simulink model "D24P414_1_model02"  (R2021a)
settings: Solver=VariableStepAuto  StartTime=0.0  StopTime=7  FixedStep=1e-6  RelTol=1e-3
values from neighbouring files (symbols this model uses):
  p_ic = climate_p    [D24P414_1_script.m]
  params_fruit = fruit_p    [D24P414_1_script.m]
  t0_shift = days(t0-t0_12_00)    [D24P414_1_script.m]
  x0_fruit = fruit_ic    [D24P414_1_script.m]
  x0_ic = climate_ic    [D24P414_1_script.m]
libraries: HORTISIM x14
(part 1 of 2)
settings Model: SimulationMode=accelerator  Creator=djoroya  LastModifiedBy=djoroya
settings SolverCC: MaxConsecutiveZCs=100  MaxConsecutiveMinStep=5
settings DebuggingCC: UnconnectedInputMsg=none  UnconnectedOutputMsg=none  UnconnectedLineMsg=none
settings HardwareCC: TargetBitPerLong=64  TargetBitPerPointer=64  TargetBitPerSizeT=64  TargetBitPerPtrDiffT=64  TargetLongLongMode=on  TargetIntDivRoundTo=Zero  TargetEndianess=LittleEndian  TargetWordSize=64  TargetHWDeviceType=MATLAB Host  ProdEqTarget=off
settings RTWCC: Description=Rapid Simulation Target  SystemTargetFile=rsim.tlc  TemplateMakefile=rsim_default_tmf
settings RSimTargetCC: TargetLangStandard=C99 (ISO)

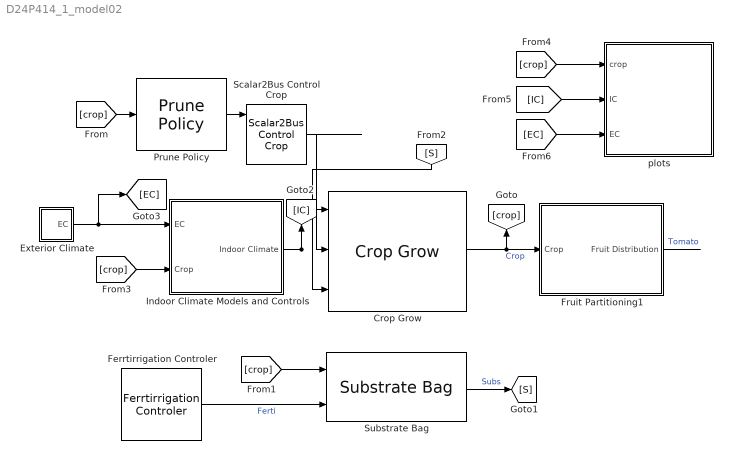
== system D24P414_1_model02 ==
  Crop Grow : HORTISIM/Horticulture/Models/Crop Grow  params=crop_params  x0=x0_crop
      settings: SourceProductName=Horti Simulator
  Exterior Climate : Subsystem
  Ferrtirrigation Controler : HORTISIM/Horticulture/Controls/Ferrtirrigation  Controler  SystemSampleTime=-1  VariantActivationTime=update diagram  Latency=0  AutoFrameSizeCalculation=off
      settings: SourceProductName=Horti Simulator
  Fruit Partitioning1 : Subsystem  AncestorBlock=HORTISIM/Horticulture/Models/Fruit Partitioning1  mask{x0=x0_fruit, params=params_fruit}
      mask Display: image('$imagefile'); % Use "Edit Image" on toolstrip to change.
  Indoor Climate Models and Controls : Subsystem
  Prune Policy : HORTISIM/Horticulture/Controls/Prune Policy  SystemSampleTime=-1  VariantActivationTime=update diagram  Latency=0  AutoFrameSizeCalculation=off
      settings: SourceProductName=Horti Simulator
  Scalar2Bus Control Crop : HORTISIM/Other  Functions/Scalar2Bus Control Crop  SystemSampleTime=-1  VariantActivationTime=update diagram  Latency=0  AutoFrameSizeCalculation=off
      settings: SourceProductName=Horti Simulator
  Substrate Bag : HORTISIM/Horticulture/Models/Substrate Bag  x0=x0_substrate  params=substrate_params
      settings: SourceProductName=Horti Simulator
  plots : Subsystem
  wires:
  Exterior Climate/1(EC) -> [EC], Indoor Climate Models and Controls/1(EC)
  Indoor Climate Models and Controls/1(Indoor Climate) -> [IC], Crop Grow/1
  Crop Grow/1 -> [crop], Fruit Partitioning1/1(Crop)  "Crop"
  Ferrtirrigation Controler/1 -> Substrate Bag/2  "Ferti"
  Scalar2Bus Control Crop/1 -> Crop Grow/2
  Prune Policy/1 -> Scalar2Bus Control Crop/1
  [crop] -> Prune Policy/1
  [crop] -> Substrate Bag/1
  Substrate Bag/1 -> [S]  "Subs"
  [S] -> Crop Grow/3
  [crop] -> Indoor Climate Models and Controls/2(Crop)
  Fruit Partitioning1/1(Fruit Distribution) -> ?  "Tomato"
  [crop] -> plots/1(crop)
  [IC] -> plots/2(IC)
  [EC] -> plots/3(EC)

== system D24P414_1_model02/Exterior Climate ==
  Demux : Demux
  From Workspace : FromWorkspace  VariableName=EC
  Scalar2Bus External Climate : HORTISIM/Other  Functions/Scalar2Bus External Climate  SystemSampleTime=-1  VariantActivationTime=update diagram  Latency=0  AutoFrameSizeCalculation=off
      settings: SourceProductName=Horti Simulator
  EC : Outport
  wires:
  Demux/3 -> Scalar2Bus External Climate/3
  Demux/2 -> Scalar2Bus External Climate/2
  Scalar2Bus External Climate/1 -> EC/1
  Demux/1 -> Scalar2Bus External Climate/1
  Demux/4 -> Scalar2Bus External Climate/4
  From Workspace/1 -> Demux/1

== system D24P414_1_model02/Fruit Partitioning1 ==
  In Bus Element : Inport  PortName=Crop  Element=Tsum
  In Bus Element1 : Inport  PortName=Crop  Element=HeatVars.TvegMean
  In Bus Element3 : Inport  PortName=Crop  Element=plants_density
  In Bus Element4 : Inport  PortName=Crop  Element=Carbon.Cfruit
  Integrator : Integrator  InitialCondition=1e-3
  MATLAB Function : MATLAB Function  TreatAsAtomicUnit=on
  Scope : Scope  NumInputPorts=2
  Scope1 : Scope
  Fruit Distribution : Outport
  wires:
  MATLAB Function/2(DT) -> Scope1/1
  In Bus Element1/1 -> MATLAB Function/4(T)
  Integrator/1 -> Scope/2, Fruit Distribution/1, MATLAB Function/3(Cfruit_mature)
  MATLAB Function/1(dCmdt) -> Integrator/1
  In Bus Element/1 -> MATLAB Function/2(Tsum)
  In Bus Element4/1 -> MATLAB Function/1(Cfruit), Scope/1

== system D24P414_1_model02/Indoor Climate Models and Controls ==
  EC : Inport
  Crop : Inport  Port=2
  Climate Model : Subsystem  Variant=on  VariantControlMode=label  VariantControl=Choice  LabelModeActiveChoice=Choice
  Control System : Subsystem
      settings: PortSchema="{\"entries\":[{\"content\":{\"sides\":[{\"content\":{\"connectorIds\":[\"In1\",\"In2\",\"In3\"]},\"type\":\"ConnectorPlacement.EquallySpacedRectSide\",\"uuid\":\"7d0146e2-a53b-49ab-a7f4-04cd7ef00b9a\"},{\"content\":{\"connectorIds\":[\"Out1\",\"Out2\"],\"side\":\"RIGHT\"},\"type\":\"ConnectorPlacement.EquallySpacedRectSide\",\"uuid\":\"fee587e2-4b5c-4140-8904-07609d427593\"},{\"content\":{\"connectorIds\":[],\"side\":\"TOP\"},\"type\":\"ConnectorPlacement.EquallySpacedRectSide\",\"uuid\":\"52e767bc-1595-40ac-996f-44c9eedd0a08\"},{\"content\":{\"connectorIds\":[\"In4\"],\"side\":\"BOTTOM\"},\"type\":\"ConnectorPlacement.EquallySpacedRectSide\",\"uuid\":\"c629db5c-cfe6-4bd1-aeb9-7fba46dde396\"}]},\"type\":\"ConnectorPlacement.EquallySpacedConnector\",\"uuid\":\"268fde01-3c08-4d62-bfbb-fc94284c5cdd\"}],\"packageUris\":[\"http://schema.mathworks.com/mf0/Connector/R2020b\"],\"version\":\"1.0\"}"
  Set Point Controler : Subsystem
      settings: PortSchema="{\"entries\":[{\"content\":{\"sides\":[{\"content\":{\"connectorIds\":[\"Out1\",\"In1\"]},\"type\":\"ConnectorPlacement.EquallySpacedRectSide\",\"uuid\":\"f4e16d49-2d4b-4271-89b5-3d9d4afc6df8\"},{\"content\":{\"connectorIds\":[],\"side\":\"RIGHT\"},\"type\":\"ConnectorPlacement.EquallySpacedRectSide\",\"uuid\":\"2cc2085b-d4b5-43d5-9499-e0c517c8a674\"},{\"content\":{\"connectorIds\":[],\"side\":\"TOP\"},\"type\":\"ConnectorPlacement.EquallySpacedRectSide\",\"uuid\":\"ad83e959-9e1e-4ed4-97a9-5adb1e75d698\"},{\"content\":{\"connectorIds\":[\"In2\"],\"side\":\"BOTTOM\"},\"type\":\"ConnectorPlacement.EquallySpacedRectSide\",\"uuid\":\"c1e716b8-742f-4738-a087-b5d9edc55981\"}]},\"type\":\"ConnectorPlacement.EquallySpacedConnector\",\"uuid\":\"8204d6bf-0a3a-4b44-b0bf-e9541e9654ff\"}],\"packageUris\":[\"http://schema.mathworks.com/mf0/Connector/R2020b\"],\"version\":\"1.0\"}"
  Indoor Climate : Outport
  wires:
  EC/1 -> Climate Model/3(EC), Control System/4(EC), Set Point Controler/2(EC)
  Crop/1 -> Control System/3(Crop), Set Point Controler/1(Crop)
  Set Point Controler/1(ST) -> Control System/2(ST)
  Control System/1(Ext) -> Climate Model/1(Ext)
  Control System/2(CoCl1) -> Climate Model/2(Control)  "Control"
  Climate Model/1(Climate) -> Control System/1(IC), Indoor Climate/1  "Indoor Climate"

== system D24P414_1_model02/plots ==
  crop : Inport
  IC : Inport  Port=2
  EC : Inport  Port=3
  Bus Selector : BusSelector  OutputSignals=Carbon.Cbuff,Carbon.Cfruit,Carbon.Cleaf,Carbon.Cstem
  Bus Selector1 : BusSelector  OutputSignals=Temp.Tair,QS.R_int
  Heater : Subsystem
  Scope : Scope  NumInputPorts=4
  Windows : Subsystem
  tag scope: R=global
  wires:
  Bus Selector/4 -> Scope/4  "<Cstem>"
  Bus Selector/3 -> Scope/3  "<Cleaf>"
  Bus Selector/2 -> Scope/2  "<Cfruit>"
  Bus Selector/1 -> Scope/1  "<Cbuff>"
  crop/1 -> Bus Selector/1
  IC/1 -> Bus Selector1/1
  Bus Selector1/2 -> [R]  "<R_int>"
  EC/1 -> Windows/1(In1), Heater/1(EC)
  Bus Selector1/1 -> Heater/2(<Tair>), Windows/2(<Tair>)  "<Tair>"

== system D24P414_1_model02/Indoor Climate Models and Controls/Climate Model ==
  Ext : Inport
  Control : Inport  Port=2
  EC : Inport  Port=3
  Climate Model : Subsystem  AncestorBlock=HORTISIM/Climate/Models/Climate Model  VariantControl=Choice  mask{params=p_ic, x0=x0_ic}
      mask Display: image('$imagefile'); % Use "Edit Image" on toolstrip to change.
  Climate : Outport

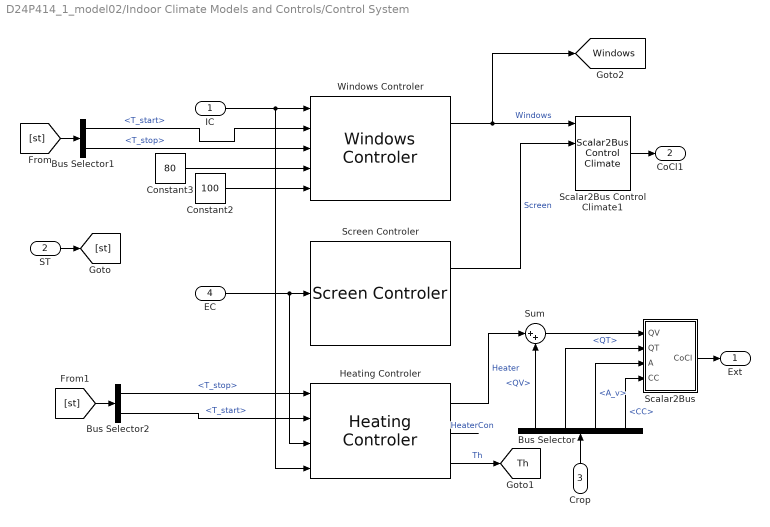
== system D24P414_1_model02/Indoor Climate Models and Controls/Control System ==
  IC : Inport
  ST : Inport  Port=2
  Crop : Inport  Port=3
  EC : Inport  Port=4
  Bus Selector : BusSelector  OutputSignals=HeatVars.QV,HeatVars.QT,A_v,CC
  Bus Selector1 : BusSelector  OutputSignals=Heater.T_start,Windows.T_stop
  Bus Selector2 : BusSelector  OutputSignals=Heater.T_stop,Heater.T_start
  Constant2 : Constant  Value=100
  Constant3 : Constant  Value=80
  Heating Controler : HORTISIM/Climate/Controls/Heating Controler  params=HP  x0=x0_H
      settings: SourceProductName=Horti Simulator
  "Scalar2Bus " : Subsystem
  Scalar2Bus Control Climate1 : HORTISIM/Other  Functions/Scalar2Bus  Control Climate  SystemSampleTime=-1  VariantActivationTime=update diagram  Latency=0  AutoFrameSizeCalculation=off
      settings: SourceProductName=Horti Simulator
  Screen Controler : HORTISIM/Climate/Controls/Screen Controler  params=scr_p
      settings: SourceProductName=Horti Simulator
  Sum : Sum  Inputs=|++
  Windows Controler : HORTISIM/Climate/Controls/Windows Controler  params=win_p
      settings: SourceProductName=Horti Simulator
  Ext : Outport
  CoCl1 : Outport  Port=2
  tag scope: Th=global, Windows=global
  wires:
  EC/1 -> Heating Controler/3, Screen Controler/1
  "Scalar2Bus "/1(CoCl) -> Ext/1
  Windows Controler/1 -> [Windows], Scalar2Bus Control Climate1/1  "Windows"
  Scalar2Bus Control Climate1/1 -> CoCl1/1
  Screen Controler/1 -> Scalar2Bus Control Climate1/2  "Screen"
  IC/1 -> Heating Controler/4, Windows Controler/1
  Constant2/1 -> Windows Controler/5
  Constant3/1 -> Windows Controler/4
  Bus Selector1/1 -> Windows Controler/2  "<T_start>"
  Bus Selector1/2 -> Windows Controler/3  "<T_stop>"
  Crop/1 -> Bus Selector/1
  Sum/1 -> "Scalar2Bus "/1(QV)
  Bus Selector/1 -> Sum/2  "<QV>"
  Heating Controler/1 -> Sum/1  "Heater"
  Bus Selector/2 -> "Scalar2Bus "/2(QT)  "<QT>"
  Bus Selector/3 -> "Scalar2Bus "/3(A)  "<A_v>"
  Bus Selector/4 -> "Scalar2Bus "/4(CC)  "<CC>"
  ST/1 -> [st]
  [st] -> Bus Selector1/1
  [st] -> Bus Selector2/1
  Heating Controler/3 -> [Th]  "Th"
  Heating Controler/2 -> ?  "HeaterCon"
  Bus Selector2/2 -> Heating Controler/2  "<T_start>"
  Bus Selector2/1 -> Heating Controler/1  "<T_stop>"

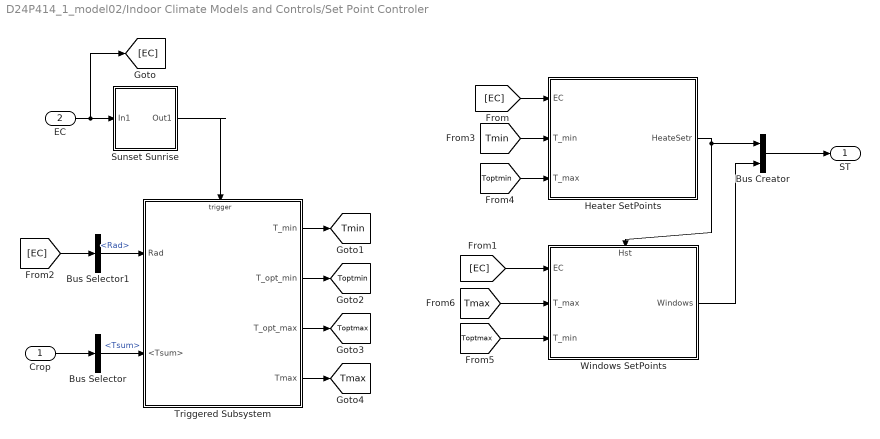
== system D24P414_1_model02/Indoor Climate Models and Controls/Set Point Controler ==
  Crop : Inport
  EC : Inport  Port=2
  Bus Creator : BusCreator  Inputs=2
  Bus Selector : BusSelector  OutputSignals=Tsum
  Bus Selector1 : BusSelector  OutputSignals=Rad
  Heater SetPoints : Subsystem
  Sunset Sunrise : Subsystem
  Triggered Subsystem : Subsystem  TreatAsAtomicUnit=on
  Windows SetPoints : Subsystem
      settings: PortSchema="{\"entries\":[{\"content\":{\"sides\":[{\"content\":{\"connectorIds\":[\"In1\",\"In2\",\"In3\"]},\"type\":\"ConnectorPlacement.EquallySpacedRectSide\",\"uuid\":\"adbf67af-74ef-4d44-a221-2fa9350c3df6\"},{\"content\":{\"connectorIds\":[\"Out1\"],\"side\":\"RIGHT\"},\"type\":\"ConnectorPlacement.EquallySpacedRectSide\",\"uuid\":\"184ab568-f69f-420e-aba1-0e27e090a144\"},{\"content\":{\"connectorIds\":[\"In4\"],\"side\":\"TOP\"},\"type\":\"ConnectorPlacement.EquallySpacedRectSide\",\"uuid\":\"ef86e682-f841-40e3-b028-22b4dc12532c\"}]},\"type\":\"ConnectorPlacement.EquallySpacedConnector\",\"uuid\":\"71dd7da4-de02-4916-9a1b-70690742187b\"}],\"packageUris\":[\"http://schema.mathworks.com/mf0/Connector/R2020b\"],\"version\":\"1.0\"}"
  ST : Outport
  tag scope: Tmax=global, Tmin=global, Toptmax=global, Toptmin=global
  wires:
  Bus Creator/1 -> ST/1
  Heater SetPoints/1(HeateSetr) -> Windows SetPoints/4(Hst), Bus Creator/1
  Windows SetPoints/1(Windows) -> Bus Creator/2
  Crop/1 -> Bus Selector/1
  Sunset Sunrise/1(Out1) -> Triggered Subsystem/Trigger
  EC/1 -> [EC], Sunset Sunrise/1(In1)
  Bus Selector/1 -> Triggered Subsystem/2(<Tsum>)  "<Tsum>"
  Bus Selector1/1 -> Triggered Subsystem/1(Rad)  "<Rad>"
  [EC] -> Heater SetPoints/1(EC)
  [EC] -> Windows SetPoints/1(EC)
  [EC] -> Bus Selector1/1
  Triggered Subsystem/2(T_opt_min) -> [Toptmin]
  Triggered Subsystem/4(Tmax) -> [Tmax]
  Triggered Subsystem/1(T_min) -> [Tmin]
  Triggered Subsystem/3(T_opt_max) -> [Toptmax]
  [Tmin] -> Heater SetPoints/2(T_min)
  [Toptmin] -> Heater SetPoints/3(T_max)
  [Toptmax] -> Windows SetPoints/3(T_min)
  [Tmax] -> Windows SetPoints/2(T_max)

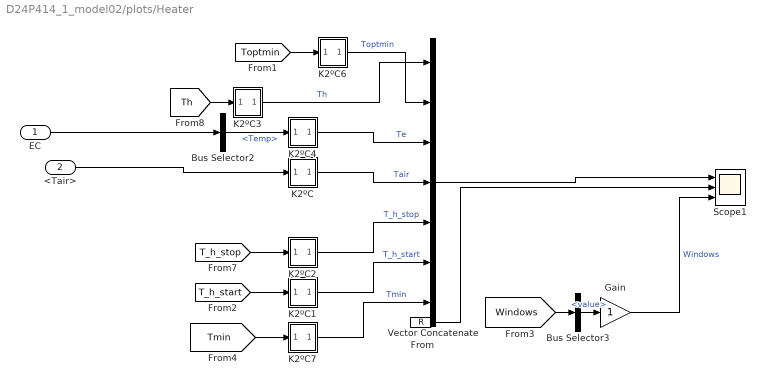
== system D24P414_1_model02/plots/Heater ==
  EC : Inport
  <Tair> : Inport  Port=2
  Bus Selector2 : BusSelector  OutputSignals=Temp
  Bus Selector3 : BusSelector  OutputSignals=value
  Gain : Gain
  K2ºC : Subsystem
  K2ºC1 : Subsystem
  K2ºC2 : Subsystem
  K2ºC3 : Subsystem
  K2ºC4 : Subsystem
  K2ºC6 : Subsystem
  K2ºC7 : Subsystem
  Scope1 : Scope  NumInputPorts=3
  Vector Concatenate : Concatenate  NumInputs=7
  wires:
  EC/1 -> Bus Selector2/1
  Bus Selector3/1 -> Gain/1  "<value>"
  [Toptmin] -> K2ºC6/1(In1)
  [R] -> Scope1/2
  K2ºC2/1(Out1) -> Vector Concatenate/5  "T_h_stop"
  Gain/1 -> Scope1/3  "Windows"
  Bus Selector2/1 -> K2ºC4/1(In1)  "<Temp>"
  K2ºC4/1(Out1) -> Vector Concatenate/3  "Te"
  [Tmin] -> K2ºC7/1(In1)
  [T_h_stop] -> K2ºC2/1(In1)
  <Tair>/1 -> K2ºC/1(In1)
  K2ºC7/1(Out1) -> Vector Concatenate/7  "Tmin"
  [Windows] -> Bus Selector3/1
  Vector Concatenate/1 -> Scope1/1
  K2ºC6/1(Out1) -> Vector Concatenate/2  "Toptmin"
  K2ºC/1(Out1) -> Vector Concatenate/4  "Tair"
  [T_h_start] -> K2ºC1/1(In1)
  K2ºC1/1(Out1) -> Vector Concatenate/6  "T_h_start"
  [Th] -> K2ºC3/1(In1)
  K2ºC3/1(Out1) -> Vector Concatenate/1  "Th"

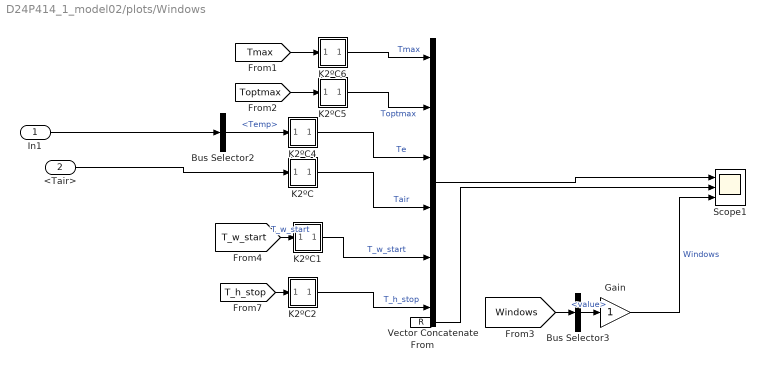
== system D24P414_1_model02/plots/Windows ==
  In1 : Inport
  <Tair> : Inport  Port=2
  Bus Selector2 : BusSelector  OutputSignals=Temp
  Bus Selector3 : BusSelector  OutputSignals=value
  Gain : Gain
  K2ºC : Subsystem
  K2ºC1 : Subsystem
  K2ºC2 : Subsystem
  K2ºC4 : Subsystem
  K2ºC5 : Subsystem
  K2ºC6 : Subsystem
  Scope1 : Scope  NumInputPorts=3
  Vector Concatenate : Concatenate  NumInputs=6
  wires:
  In1/1 -> Bus Selector2/1
  Bus Selector3/1 -> Gain/1  "<value>"
  [Toptmax] -> K2ºC5/1(In1)
  [Tmax] -> K2ºC6/1(In1)
  [R] -> Scope1/2
  K2ºC2/1(Out1) -> Vector Concatenate/6  "T_h_stop"
  K2ºC5/1(Out1) -> Vector Concatenate/2  "Toptmax"
  Gain/1 -> Scope1/3  "Windows"
  Bus Selector2/1 -> K2ºC4/1(In1)  "<Temp>"
  K2ºC4/1(Out1) -> Vector Concatenate/3  "Te"
  [T_h_stop] -> K2ºC2/1(In1)
  <Tair>/1 -> K2ºC/1(In1)
  [Windows] -> Bus Selector3/1
  Vector Concatenate/1 -> Scope1/1
  K2ºC6/1(Out1) -> Vector Concatenate/1  "Tmax"
  K2ºC/1(Out1) -> Vector Concatenate/4  "Tair"
  K2ºC1/1(Out1) -> Vector Concatenate/5  "T_w_start"
  [T_w_start] -> K2ºC1/1(In1)  "T_w_start"

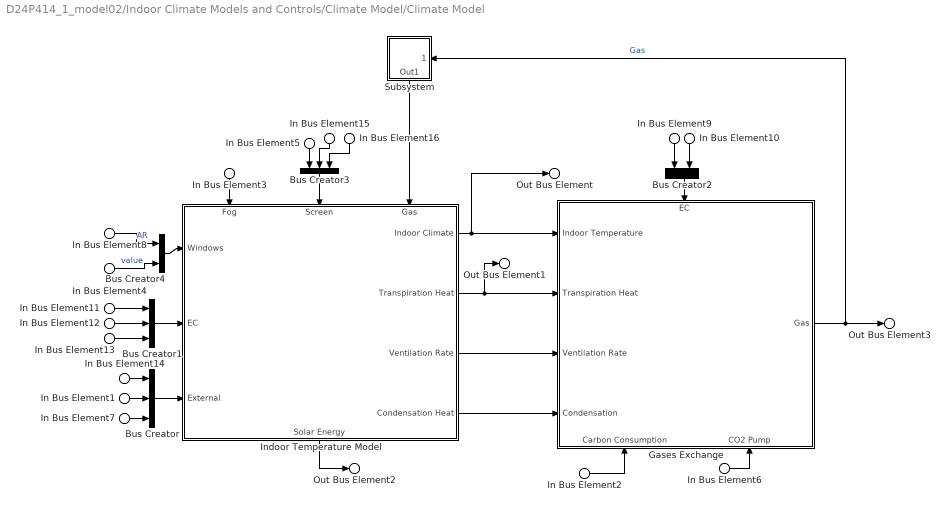
== system D24P414_1_model02/Indoor Climate Models and Controls/Climate Model/Climate Model ==
  In Bus Element14 : Inport  PortName=Ext  Element=QT
  In Bus Element1 : Inport  PortName=Ext  Element=QV
  In Bus Element2 : Inport  PortName=Ext  Element=CC
  In Bus Element7 : Inport  PortName=Ext  Element=A
  In Bus Element3 : Inport  Port=2  PortName=Control  Element=Fog
  In Bus Element5 : Inport  Port=2  PortName=Control  Element=Screen.gamma_max
  In Bus Element15 : Inport  Port=2  PortName=Control  Element=Screen.value
  In Bus Element16 : Inport  Port=2  PortName=Control  Element=Screen.beta
  In Bus Element6 : Inport  Port=2  PortName=Control  Element=CO2
  In Bus Element8 : Inport  Port=2  PortName=Control  Element=Windows.AR
  In Bus Element4 : Inport  Port=2  PortName=Control  Element=Windows.value
  In Bus Element9 : Inport  Port=3  PortName=EC  Element=HR
  In Bus Element10 : Inport  Port=3  PortName=EC  Element=Temp
  In Bus Element11 : Inport  Port=3  PortName=EC  Element=Temp
  In Bus Element12 : Inport  Port=3  PortName=EC  Element=Rad
  In Bus Element13 : Inport  Port=3  PortName=EC  Element=Wind
  Bus Creator : BusCreator  Inputs=3
  Bus Creator1 : BusCreator  Inputs=3
  Bus Creator2 : BusCreator  Inputs=2
  Bus Creator3 : BusCreator  Inputs=3
  Bus Creator4 : BusCreator  Inputs=2
  Gases Exchange : Subsystem
      settings: PortSchema="{\"entries\":[{\"content\":{\"sides\":[{\"content\":{\"connectorIds\":[\"In1\",\"In2\",\"In3\",\"In4\"]},\"type\":\"ConnectorPlacement.EquallySpacedRectSide\",\"uuid\":\"550da9a1-5f22-4db3-9ee3-e3750278f626\"},{\"content\":{\"connectorIds\":[\"Out1\"],\"side\":\"RIGHT\"},\"type\":\"ConnectorPlacement.EquallySpacedRectSide\",\"uuid\":\"cf559ec0-337d-42e7-96bb-a49ff9e682f6\"},{\"content\":{\"connectorIds\":[\"In5\"],\"side\":\"TOP\"},\"type\":\"ConnectorPlacement.EquallySpacedRectSide\",\"uuid\":\"d9874986-c35c-443c-9325-7a886074565b\"},{\"content\":{\"connectorIds\":[\"In6\",\"In7\"],\"side\":\"BOTTOM\"},\"type\":\"ConnectorPlacement.EquallySpacedRectSide\",\"uuid\":\"7f205c84-db2c-43a4-94ce-a6d2142a4e50\"}]},\"type\":\"ConnectorPlacement.EquallySpacedConnector\",\"uuid\":\"56c5cbc1-f580-43fc-9d79-62500ce9be4b\"}],\"packageUris\":[\"http://schema.mathworks.com/mf0/Connector/R2020b\"],\"version\":\"1.0\"}"
  Indoor Temperature Model : Subsystem
      settings: PortSchema="{\"entries\":[{\"content\":{\"sides\":[{\"content\":{\"connectorIds\":[\"In1\",\"In2\",\"In3\"]},\"type\":\"ConnectorPlacement.EquallySpacedRectSide\",\"uuid\":\"402556d7-b277-4cb3-8556-883bae99c69c\"},{\"content\":{\"connectorIds\":[\"Out1\",\"Out2\",\"Out3\",\"Out4\"],\"side\":\"RIGHT\"},\"type\":\"ConnectorPlacement.EquallySpacedRectSide\",\"uuid\":\"e8ec9f82-8759-4d98-a5e5-ef4db996ec8c\"},{\"content\":{\"connectorIds\":[\"In4\",\"In5\",\"In6\"],\"side\":\"TOP\"},\"type\":\"ConnectorPlacement.EquallySpacedRectSide\",\"uuid\":\"99d33cea-a089-4bcb-9505-68914c63f152\"},{\"content\":{\"connectorIds\":[\"Out5\"],\"side\":\"BOTTOM\"},\"type\":\"ConnectorPlacement.EquallySpacedRectSide\",\"uuid\":\"61ead6b3-0464-47f9-9f23-19f86056b325\"}]},\"type\":\"ConnectorPlacement.EquallySpacedConnector\",\"uuid\":\"a07dfd2f-7b40-4439-87f5-f093ac984b26\"}],\"packageUris\":[\"http://schema.mathworks.com/mf0/Connector/R2020b\"],\"version\":\"1.0\"}"
  Subsystem : Subsystem
      settings: PortSchema="{\"entries\":[{\"content\":{\"sides\":[{\"content\":{\"connectorIds\":[]},\"type\":\"ConnectorPlacement.EquallySpacedRectSide\",\"uuid\":\"35868875-f783-4ad4-af7a-8ba6d23e35d0\"},{\"content\":{\"connectorIds\":[\"Out1\"],\"side\":\"RIGHT\"},\"type\":\"ConnectorPlacement.EquallySpacedRectSide\",\"uuid\":\"2025d12d-e021-4399-bfe6-d7037c727539\"},{\"content\":{\"connectorIds\":[],\"side\":\"TOP\"},\"type\":\"ConnectorPlacement.EquallySpacedRectSide\",\"uuid\":\"3e424627-322e-4117-9014-21364a52cbdc\"},{\"content\":{\"connectorIds\":[\"In1\"],\"side\":\"BOTTOM\"},\"type\":\"ConnectorPlacement.EquallySpacedRectSide\",\"uuid\":\"db7a2526-7ee4-413d-8e1d-de852bb4cdfb\"}]},\"type\":\"ConnectorPlacement.EquallySpacedConnector\",\"uuid\":\"c6534136-4261-4144-9645-4fbbe9dd779a\"}],\"packageUris\":[\"http://schema.mathworks.com/mf0/Connector/R2020b\"],\"version\":\"1.0\"}"
  Out Bus Element : Outport  PortName=Climate  Element=Temp
  Out Bus Element1 : Outport  PortName=Climate  Element=QT
  Out Bus Element2 : Outport  PortName=Climate  Element=QS
  Out Bus Element3 : Outport  PortName=Climate  Element=Gas
  wires:
  In Bus Element7/1 -> Bus Creator/3
  Bus Creator/1 -> Indoor Temperature Model/3(External)
  In Bus Element14/1 -> Bus Creator/1
  In Bus Element1/1 -> Bus Creator/2
  In Bus Element10/1 -> Bus Creator2/2
  In Bus Element9/1 -> Bus Creator2/1
  Bus Creator2/1 -> Gases Exchange/5(EC)
  Bus Creator1/1 -> Indoor Temperature Model/2(EC)
  In Bus Element11/1 -> Bus Creator1/1
  In Bus Element13/1 -> Bus Creator1/3
  In Bus Element12/1 -> Bus Creator1/2
  In Bus Element6/1 -> Gases Exchange/7(CO2 Pump)
  In Bus Element3/1 -> Indoor Temperature Model/4(Fog)
  Indoor Temperature Model/5(Solar Energy) -> Out Bus Element2/1
  Indoor Temperature Model/2(Transpiration Heat) -> Out Bus Element1/1, Gases Exchange/2(Transpiration Heat)
  Indoor Temperature Model/1(Indoor Climate) -> Gases Exchange/1(Indoor Temperature), Out Bus Element/1
  Indoor Temperature Model/3(Ventilation Rate) -> Gases Exchange/3(Ventilation Rate)
  Indoor Temperature Model/4(Condensation Heat) -> Gases Exchange/4(Condensation)
  In Bus Element2/1 -> Gases Exchange/6(Carbon Consumption)
  Gases Exchange/1(" Gas") -> Subsystem/1(Gas), Out Bus Element3/1  "Gas"
  In Bus Element4/1 -> Bus Creator4/2  "value"
  In Bus Element8/1 -> Bus Creator4/1  "AR"
  Bus Creator4/1 -> Indoor Temperature Model/1(Windows)
  Subsystem/1(Out1) -> Indoor Temperature Model/6(Gas)
  Bus Creator3/1 -> Indoor Temperature Model/5(Screen)
  In Bus Element5/1 -> Bus Creator3/1
  In Bus Element15/1 -> Bus Creator3/2
  In Bus Element16/1 -> Bus Creator3/3

== system D24P414_1_model02/Indoor Climate Models and Controls/Control System/Scalar2Bus  ==
  QV : Inport
  QT : Inport  Port=2
  A : Inport  Port=3
  CC : Inport  Port=4
  Bus Creator : BusCreator  Inputs=4
  CoCl : Outport
  wires:
  A/1 -> Bus Creator/3  "A"
  CC/1 -> Bus Creator/4  "CC"
  QV/1 -> Bus Creator/1  "QV"
  Bus Creator/1 -> CoCl/1
  QT/1 -> Bus Creator/2  "QT"

== system D24P414_1_model02/Indoor Climate Models and Controls/Set Point Controler/Heater SetPoints ==
  EC : Inport
  T_min : Inport  Port=2
  T_max : Inport  Port=3
  Bus Creator1 : BusCreator  Inputs=2
  Bus Selector2 : BusSelector  OutputSignals=Temp
  Subsystem1 : Subsystem
  HeateSetr : Outport
  tag scope: T_h_start=global, T_h_stop=global
  wires:
  Subsystem1/1(T_start) -> [T_h_start], Bus Creator1/1  "T_start"
  EC/1 -> Bus Selector2/1
  Bus Creator1/1 -> HeateSetr/1  "Heater"
  Bus Selector2/1 -> Subsystem1/3(<Temp>)  "<Temp>"
  Subsystem1/2(T_stop) -> [T_h_stop], Bus Creator1/2  "T_stop"
  T_min/1 -> Subsystem1/1(T_min)
  T_max/1 -> Subsystem1/2(T_max)

== system D24P414_1_model02/Indoor Climate Models and Controls/Set Point Controler/Sunset Sunrise ==
  In1 : Inport
  Bus Selector : BusSelector  OutputSignals=Rad
  Constant4 : Constant  Value=100
  Gain : Gain  Gain=10
  Minus : Sum  Inputs=+-
  Tan : Trigonometry  Operator=tanh
  Out1 : Outport
  wires:
  In1/1 -> Bus Selector/1
  Constant4/1 -> Minus/2
  Tan/1 -> Out1/1
  Gain/1 -> Tan/1
  Minus/1 -> Gain/1
  Bus Selector/1 -> Minus/1  "<Rad>"

== system D24P414_1_model02/Indoor Climate Models and Controls/Set Point Controler/Triggered Subsystem ==
  Rad : Inport
  <Tsum> : Inport  Port=2
  Trigger : TriggerPort  TriggerType=either  VariantControl=(inherit)  InitialTriggerSignalState=positive
  Constant : Constant  Value=100
  MATLAB Function : MATLAB Function  TreatAsAtomicUnit=on
  T_min : Outport
  T_opt_min : Outport  Port=2
  T_opt_max : Outport  Port=3
  Tmax : Outport  Port=4
  wires:
  <Tsum>/1 -> MATLAB Function/1(Tsum)
  Rad/1 -> MATLAB Function/2(Rad)
  Constant/1 -> MATLAB Function/3(THRad)
  MATLAB Function/1(T_min) -> T_min/1
  MATLAB Function/2(T_opt_min) -> T_opt_min/1
  MATLAB Function/3(T_opt_max) -> T_opt_max/1
  MATLAB Function/4(Tmax) -> Tmax/1

== system D24P414_1_model02/Indoor Climate Models and Controls/Set Point Controler/Windows SetPoints ==
  EC : Inport
  T_max : Inport  Port=2
  T_min : Inport  Port=3
  Hst : Inport  Port=4
  Bus Creator2 : BusCreator  Inputs=2
  Bus Selector1 : BusSelector  OutputSignals=T_stop
  Constant : Constant  Value=10
  Constant1 : Constant
  Sum : Sum  Inputs=|++
  Sum1 : Sum  Inputs=|++
  Windows : Outport
  tag scope: T_w_start=global, T_w_stop=global
  wires:
  Bus Creator2/1 -> Windows/1  "Windows"
  Sum/1 -> [T_w_stop], Bus Creator2/2  "T_stop"
  T_min/1 -> Sum1/1  "T_start"
  Constant/1 -> Sum/1
  Hst/1 -> Bus Selector1/1
  Constant1/1 -> Sum1/2
  Sum1/1 -> Bus Creator2/1, Sum/2, [T_w_start]

== system D24P414_1_model02/plots/Heater/K2ºC ==
  In1 : Inport
  Constant : Constant  Value=273.15
  Minus : Sum  Inputs=+-
  Out1 : Outport
  wires:
  Minus/1 -> Out1/1
  In1/1 -> Minus/1
  Constant/1 -> Minus/2

== system D24P414_1_model02/plots/Heater/K2ºC1 ==
  In1 : Inport
  Constant : Constant  Value=273.15
  Minus : Sum  Inputs=+-
  Out1 : Outport
  wires:
  Minus/1 -> Out1/1
  In1/1 -> Minus/1
  Constant/1 -> Minus/2

== system D24P414_1_model02/plots/Heater/K2ºC2 ==
  In1 : Inport
  Constant : Constant  Value=273.15
  Minus : Sum  Inputs=+-
  Out1 : Outport
  wires:
  Minus/1 -> Out1/1
  In1/1 -> Minus/1
  Constant/1 -> Minus/2

== system D24P414_1_model02/plots/Heater/K2ºC3 ==
  In1 : Inport
  Constant : Constant  Value=273.15
  Minus : Sum  Inputs=+-
  Out1 : Outport
  wires:
  Minus/1 -> Out1/1
  In1/1 -> Minus/1
  Constant/1 -> Minus/2

== system D24P414_1_model02/plots/Heater/K2ºC4 ==
  In1 : Inport
  Constant : Constant  Value=273.15
  Minus : Sum  Inputs=+-
  Out1 : Outport
  wires:
  Minus/1 -> Out1/1
  In1/1 -> Minus/1
  Constant/1 -> Minus/2

== system D24P414_1_model02/plots/Heater/K2ºC6 ==
  In1 : Inport
  Constant : Constant  Value=273.15
  Minus : Sum  Inputs=+-
  Out1 : Outport
  wires:
  Minus/1 -> Out1/1
  In1/1 -> Minus/1
  Constant/1 -> Minus/2

== system D24P414_1_model02/plots/Heater/K2ºC7 ==
  In1 : Inport
  Constant : Constant  Value=273.15
  Minus : Sum  Inputs=+-
  Out1 : Outport
  wires:
  Minus/1 -> Out1/1
  In1/1 -> Minus/1
  Constant/1 -> Minus/2

== system D24P414_1_model02/plots/Windows/K2ºC ==
  In1 : Inport
  Constant : Constant  Value=273.15
  Minus : Sum  Inputs=+-
  Out1 : Outport
  wires:
  Minus/1 -> Out1/1
  In1/1 -> Minus/1
  Constant/1 -> Minus/2

== system D24P414_1_model02/plots/Windows/K2ºC1 ==
  In1 : Inport
  Constant : Constant  Value=273.15
  Minus : Sum  Inputs=+-
  Out1 : Outport
  wires:
  Minus/1 -> Out1/1
  In1/1 -> Minus/1
  Constant/1 -> Minus/2

== system D24P414_1_model02/plots/Windows/K2ºC2 ==
  In1 : Inport
  Constant : Constant  Value=273.15
  Minus : Sum  Inputs=+-
  Out1 : Outport
  wires:
  Minus/1 -> Out1/1
  In1/1 -> Minus/1
  Constant/1 -> Minus/2

== system D24P414_1_model02/plots/Windows/K2ºC4 ==
  In1 : Inport
  Constant : Constant  Value=273.15
  Minus : Sum  Inputs=+-
  Out1 : Outport
  wires:
  Minus/1 -> Out1/1
  In1/1 -> Minus/1
  Constant/1 -> Minus/2

== system D24P414_1_model02/plots/Windows/K2ºC5 ==
  In1 : Inport
  Constant : Constant  Value=273.15
  Minus : Sum  Inputs=+-
  Out1 : Outport
  wires:
  Minus/1 -> Out1/1
  In1/1 -> Minus/1
  Constant/1 -> Minus/2

== system D24P414_1_model02/plots/Windows/K2ºC6 ==
  In1 : Inport
  Constant : Constant  Value=273.15
  Minus : Sum  Inputs=+-
  Out1 : Outport
  wires:
  Minus/1 -> Out1/1
  In1/1 -> Minus/1
  Constant/1 -> Minus/2

== system D24P414_1_model02/Indoor Climate Models and Controls/Climate Model/Climate Model/Gases Exchange ==
  Indoor Temperature : Inport
  Transpiration Heat : Inport  Port=2
  Ventilation Rate : Inport  Port=3
  Condensation : Inport  Port=4
  In Bus Element : Inport  Port=5  PortName=EC  Element=Temp
  In Bus Element1 : Inport  Port=5  PortName=EC  Element=HR
  Carbon Consumption : Inport  Port=6
  CO2 Pump : Inport  Port=7
  Carbon Dynamics : Subsystem
      settings: PortSchema="{\"entries\":[{\"content\":{\"sides\":[{\"content\":{\"connectorIds\":[\"In1\",\"In2\",\"In3\"]},\"type\":\"ConnectorPlacement.EquallySpacedRectSide\",\"uuid\":\"ce6da3e3-21f1-4394-8848-c3b9ed37cfe4\"},{\"content\":{\"connectorIds\":[\"Out1\",\"Out2\"],\"side\":\"RIGHT\"},\"type\":\"ConnectorPlacement.EquallySpacedRectSide\",\"uuid\":\"ff9d1dc7-ad1d-4f02-8424-55a857bc099f\"},{\"content\":{\"connectorIds\":[\"In4\",\"In5\"],\"side\":\"TOP\"},\"type\":\"ConnectorPlacement.EquallySpacedRectSide\",\"uuid\":\"728a06d8-4ce2-49f0-80dc-b6302b266d7a\"}]},\"type\":\"ConnectorPlacement.EquallySpacedConnector\",\"uuid\":\"a07ea8b7-add0-4d37-8d5e-856da5f5b640\"}],\"packageUris\":[\"http://schema.mathworks.com/mf0/Connector/R2020b\"],\"version\":\"1.0\"}"
  Compute Mid Variables : Subsystem
      settings: PortSchema="{\"entries\":[{\"content\":{\"sides\":[{\"content\":{\"connectorIds\":[\"In1\",\"In2\"]},\"type\":\"ConnectorPlacement.EquallySpacedRectSide\",\"uuid\":\"c9e251e2-f19d-4856-b15c-3b9f1eb64f83\"},{\"content\":{\"connectorIds\":[\"Out1\"],\"side\":\"RIGHT\"},\"type\":\"ConnectorPlacement.EquallySpacedRectSide\",\"uuid\":\"10734817-c937-42fb-8ae5-9505620c6f0f\"},{\"content\":{\"connectorIds\":[],\"side\":\"TOP\"},\"type\":\"ConnectorPlacement.EquallySpacedRectSide\",\"uuid\":\"8c056440-d8bf-4ff4-85aa-0f6a5eb7f23f\"},{\"content\":{\"connectorIds\":[\"In3\"],\"side\":\"BOTTOM\"},\"type\":\"ConnectorPlacement.EquallySpacedRectSide\",\"uuid\":\"fc2511c5-58d6-455e-9438-4abf6bda86a2\"}]},\"type\":\"ConnectorPlacement.EquallySpacedConnector\",\"uuid\":\"13e72cfa-9d8f-4756-adac-f24fb0238c2a\"}],\"packageUris\":[\"http://schema.mathworks.com/mf0/Connector/R2020b\"],\"version\":\"1.0\"}"
  Gain1 : Gain  Gain=24*3600
  Integrator1 : Integrator  InitialCondition=x0.G0  AbsoluteTolerance=1e-5
  Vector Concatenate : Concatenate
  Water Dynamics : Subsystem
      settings: PortSchema="{\"entries\":[{\"content\":{\"sides\":[{\"content\":{\"connectorIds\":[\"In1\",\"In2\",\"In3\"]},\"type\":\"ConnectorPlacement.EquallySpacedRectSide\",\"uuid\":\"ce6da3e3-21f1-4394-8848-c3b9ed37cfe4\"},{\"content\":{\"connectorIds\":[\"Out1\"],\"side\":\"RIGHT\"},\"type\":\"ConnectorPlacement.EquallySpacedRectSide\",\"uuid\":\"ff9d1dc7-ad1d-4f02-8424-55a857bc099f\"},{\"content\":{\"connectorIds\":[\"In4\"],\"side\":\"TOP\"},\"type\":\"ConnectorPlacement.EquallySpacedRectSide\",\"uuid\":\"728a06d8-4ce2-49f0-80dc-b6302b266d7a\"},{\"content\":{\"connectorIds\":[\"In5\",\"In6\"],\"side\":\"BOTTOM\"},\"type\":\"ConnectorPlacement.EquallySpacedRectSide\",\"uuid\":\"cc1d9c53-b6c6-41b0-b878-c109c9de6d5f\"}]},\"type\":\"ConnectorPlacement.EquallySpacedConnector\",\"uuid\":\"a07ea8b7-add0-4d37-8d5e-856da5f5b640\"}],\"packageUris\":[\"http://schema.mathworks.com/mf0/Connector/R2020b\"],\"version\":\"1.0\"}"
  " Gas" : Outport
  wires:
  Carbon Dynamics/2(C_ce) -> Compute Mid Variables/3(C_ce)
  In Bus Element1/1 -> Water Dynamics/4(He)
  In Bus Element/1 -> Water Dynamics/5(Te), Carbon Dynamics/4(Te)
  CO2 Pump/1 -> Carbon Dynamics/2(MC_cc_i)
  Condensation/1 -> Water Dynamics/3(Condensation)
  Compute Mid Variables/1(Gas) -> " Gas"/1, Carbon Dynamics/3(GasComp), Water Dynamics/1(GasComp)
  Indoor Temperature/1 -> Compute Mid Variables/2(Indoor Temperature)
  Ventilation Rate/1 -> Water Dynamics/6(Ventilation Rate), Carbon Dynamics/5(Ventilation Rate)
  Carbon Dynamics/1(dC_c_dt) -> Vector Concatenate/2
  Carbon Consumption/1 -> Carbon Dynamics/1(CarbonC)
  Water Dynamics/1(dC_w_dt) -> Vector Concatenate/1
  Transpiration Heat/1 -> Water Dynamics/2(Latent Heat)
  Integrator1/1 -> Compute Mid Variables/1(Gas_Conc)
  Vector Concatenate/1 -> Gain1/1
  Gain1/1 -> Integrator1/1

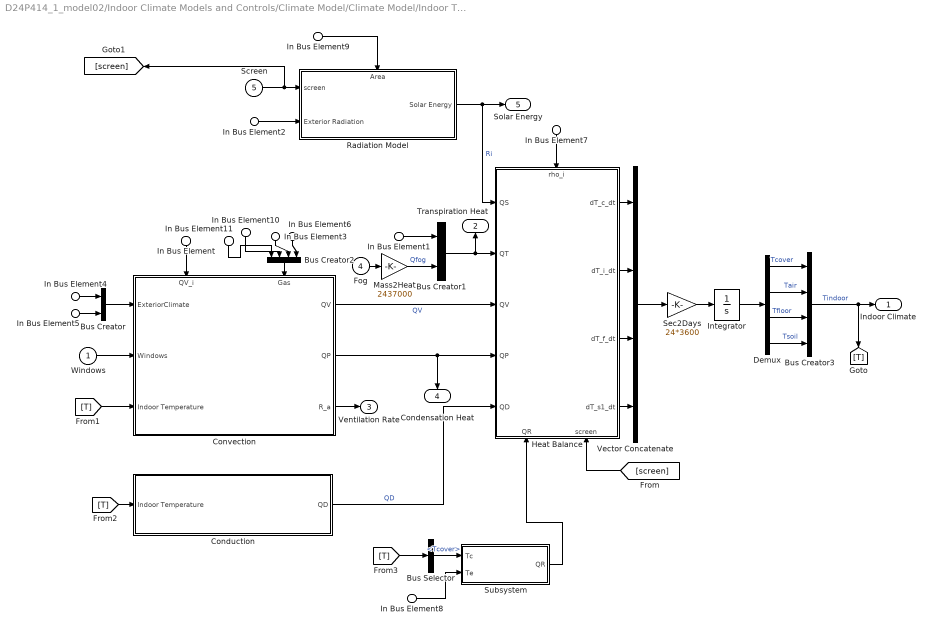
== system D24P414_1_model02/Indoor Climate Models and Controls/Climate Model/Climate Model/Indoor Temperature Model ==
  Windows : Inport
  In Bus Element2 : Inport  Port=2  PortName=EC  Element=Rad
  In Bus Element4 : Inport  Port=2  PortName=EC  Element=Temp
  In Bus Element8 : Inport  Port=2  PortName=EC  Element=Temp
  In Bus Element5 : Inport  Port=2  PortName=EC  Element=Wind
  In Bus Element : Inport  Port=3  PortName=External  Element=QV
  In Bus Element1 : Inport  Port=3  PortName=External  Element=QT
  In Bus Element9 : Inport  Port=3  PortName=External  Element=A
  Fog : Inport  Port=4
  Screen : Inport  Port=5
  In Bus Element3 : Inport  Port=6  PortName=Gas  Element=C_w
  In Bus Element6 : Inport  Port=6  PortName=Gas  Element=rho_i
  In Bus Element7 : Inport  Port=6  PortName=Gas  Element=rho_i
  In Bus Element10 : Inport  Port=6  PortName=Gas  Element=C_w_sat_T_c
  In Bus Element11 : Inport  Port=6  PortName=Gas  Element=C_w_sat_T_f
  Bus Creator : BusCreator  Inputs=2
  Bus Creator1 : BusCreator  Inputs=2
  Bus Creator2 : BusCreator  Inputs=4
  Bus Creator3 : BusCreator  Inputs=4
  Bus Selector : BusSelector  OutputSignals=Tcover
  Conduction : Subsystem
  Convection : Subsystem
      settings: PortSchema="{\"entries\":[{\"content\":{\"sides\":[{\"content\":{\"connectorIds\":[\"In1\",\"In2\",\"In3\"]},\"type\":\"ConnectorPlacement.EquallySpacedRectSide\",\"uuid\":\"3a7e199a-659d-4634-89e1-ef85cb7ed502\"},{\"content\":{\"connectorIds\":[\"Out1\",\"Out2\",\"Out3\"],\"side\":\"RIGHT\"},\"type\":\"ConnectorPlacement.EquallySpacedRectSide\",\"uuid\":\"10ed7806-8be5-4e88-a0ca-6abfb5c9ab8d\"},{\"content\":{\"connectorIds\":[\"In4\",\"In5\"],\"side\":\"TOP\"},\"type\":\"ConnectorPlacement.EquallySpacedRectSide\",\"uuid\":\"907defe4-ff8f-4a74-ba27-620529c27b74\"},{\"content\":{\"connectorIds\":[],\"side\":\"BOTTOM\"},\"type\":\"ConnectorPlacement.EquallySpacedRectSide\",\"uuid\":\"397bdb42-e8ee-4be9-8569-3130f6cbf999\"}]},\"type\":\"ConnectorPlacement.EquallySpacedConnector\",\"uuid\":\"f437f85f-61b6-4f41-a544-29e333cf1086\"}],\"packageUris\":[\"http://schema.mathworks.com/mf0/Connector/R2020b\"],\"version\":\"1.0\"}"
  Demux : Demux
  Heat Balance : Subsystem
      settings: PortSchema="{\"entries\":[{\"content\":{\"sides\":[{\"content\":{\"connectorIds\":[\"In1\",\"In2\",\"In3\",\"In4\",\"In5\"]},\"type\":\"ConnectorPlacement.EquallySpacedRectSide\",\"uuid\":\"ccfbb954-e9e7-4841-9dc1-a760315eb250\"},{\"content\":{\"connectorIds\":[\"Out1\",\"Out2\",\"Out3\",\"Out4\"],\"side\":\"RIGHT\"},\"type\":\"ConnectorPlacement.EquallySpacedRectSide\",\"uuid\":\"e9754eb2-54ce-43cf-bf33-7cf2f1345c42\"},{\"content\":{\"connectorIds\":[\"In6\"],\"side\":\"TOP\"},\"type\":\"ConnectorPlacement.EquallySpacedRectSide\",\"uuid\":\"6ccd5de1-b6bb-47c5-ac6c-9382e354fee6\"},{\"content\":{\"connectorIds\":[\"In7\",\"In8\"],\"side\":\"BOTTOM\"},\"type\":\"ConnectorPlacement.EquallySpacedRectSide\",\"uuid\":\"dba41702-708c-4231-8998-8d54661f4881\"}]},\"type\":\"ConnectorPlacement.EquallySpacedConnector\",\"uuid\":\"31920c9d-5e0f-4503-9ddd-ce99d792a3e0\"}],\"packageUris\":[\"http://schema.mathworks.com/mf0/Connector/R2020b\"],\"version\":\"1.0\"}"
  Integrator : Integrator  InitialCondition=x0.T0  AbsoluteTolerance=0.01
  Mass2Heat : Gain  Gain=2437000
  Radiation Model : Subsystem
      settings: PortSchema="{\"entries\":[{\"content\":{\"sides\":[{\"content\":{\"connectorIds\":[\"In1\",\"In2\"]},\"type\":\"ConnectorPlacement.EquallySpacedRectSide\",\"uuid\":\"cb5a2538-07d5-409a-bc47-ac7157db0ef4\"},{\"content\":{\"connectorIds\":[\"Out1\"],\"side\":\"RIGHT\"},\"type\":\"ConnectorPlacement.EquallySpacedRectSide\",\"uuid\":\"7dfe2e6f-8ee6-45c0-8502-080571e1b483\"},{\"content\":{\"connectorIds\":[\"In3\"],\"side\":\"TOP\"},\"type\":\"ConnectorPlacement.EquallySpacedRectSide\",\"uuid\":\"52df64bb-9cf1-44e4-8c24-fa6c372d73f1\"}]},\"type\":\"ConnectorPlacement.EquallySpacedConnector\",\"uuid\":\"b803895f-b114-4368-b273-36a7794022b5\"}],\"packageUris\":[\"http://schema.mathworks.com/mf0/Connector/R2020b\"],\"version\":\"1.0\"}"
  Sec2Days : Gain  Gain=24*3600
  Subsystem : Subsystem
  Vector Concatenate : Concatenate  NumInputs=4
  Indoor Climate : Outport
  Transpiration Heat : Outport  Port=2
  Ventilation Rate : Outport  Port=3
  Condensation Heat : Outport  Port=4
  Solar Energy : Outport  Port=5
  wires:
  In Bus Element11/1 -> Bus Creator2/1
  In Bus Element10/1 -> Bus Creator2/2
  In Bus Element9/1 -> Radiation Model/3(Area)
  Subsystem/1(QR) -> Heat Balance/7(QR)
  Bus Selector/1 -> Subsystem/1(Tc)  "<Tcover>"
  [T] -> Bus Selector/1
  In Bus Element8/1 -> Subsystem/2(Te)
  Integrator/1 -> Demux/1
  Demux/1 -> Bus Creator3/1  "Tcover"
  Demux/2 -> Bus Creator3/2  "Tair"
  Demux/3 -> Bus Creator3/3  "Tfloor"
  Demux/4 -> Bus Creator3/4  "Tsoil"
  Bus Creator3/1 -> Indoor Climate/1, [T]  "Tindoor"
  In Bus Element/1 -> Convection/4(QV_i)
  In Bus Element6/1 -> Bus Creator2/4
  In Bus Element3/1 -> Bus Creator2/3
  Bus Creator2/1 -> Convection/5(Gas)
  Bus Creator1/1 -> Transpiration Heat/1, Heat Balance/2(QT)
  In Bus Element1/1 -> Bus Creator1/1
  Mass2Heat/1 -> Bus Creator1/2  "Qfog"
  Fog/1 -> Mass2Heat/1
  In Bus Element5/1 -> Bus Creator/2
  In Bus Element4/1 -> Bus Creator/1
  Screen/1 -> [screen], Radiation Model/1(screen)
  Bus Creator/1 -> Convection/1(ExteriorClimate)
  Radiation Model/1("Solar Energy  ") -> Heat Balance/1(QS), Solar Energy/1  "Ri"
  In Bus Element2/1 -> Radiation Model/2(Exterior Radiation)
  Windows/1 -> Convection/2(Windows)
  Convection/2(QP) -> Heat Balance/4(QP), Condensation Heat/1
  In Bus Element7/1 -> Heat Balance/6(rho_i)
  [T] -> Conduction/1(Indoor Temperature)
  [T] -> Convection/3(Indoor Temperature)
  Heat Balance/1(dT_c_dt) -> Vector Concatenate/1
  Heat Balance/4(dT_s1_dt) -> Vector Concatenate/4
  Heat Balance/3(dT_f_dt) -> Vector Concatenate/3
  Heat Balance/2(dT_i_dt) -> Vector Concatenate/2
  Conduction/1(QD) -> Heat Balance/5(QD)  "QD"
  Convection/1(QV) -> Heat Balance/3(QV)  "QV"
  Convection/3(R_a) -> Ventilation Rate/1
  Sec2Days/1 -> Integrator/1
  Vector Concatenate/1 -> Sec2Days/1
  [screen] -> Heat Balance/8(screen)

== system D24P414_1_model02/Indoor Climate Models and Controls/Climate Model/Climate Model/Subsystem ==
  Gas : Inport
  Bus Creator3 : BusCreator  Inputs=4
  Bus Selector : BusSelector  OutputSignals=C_w,rho_i,C_w_sat_T_c,C_w_sat_T_f
  Out1 : Outport
  wires:
  Gas/1 -> Bus Selector/1
  Bus Selector/4 -> Bus Creator3/4  "<C_w_sat_T_f>"
  Bus Selector/2 -> Bus Creator3/2  "<rho_i>"
  Bus Selector/1 -> Bus Creator3/1  "<C_w>"
  Bus Creator3/1 -> Out1/1
  Bus Selector/3 -> Bus Creator3/3  "<C_w_sat_T_c>"

== system D24P414_1_model02/Indoor Climate Models and Controls/Set Point Controler/Heater SetPoints/Subsystem1 ==
  T_min : Inport
  T_max : Inport  Port=2
  <Temp> : Inport  Port=3
  Constant : Constant  Value=2
  Every Day : Subsystem
  Every Day1 : Subsystem
  If : If  IfExpression=u1 == 1  ElseIfExpressions=u1 == 2,u1 == 3,u1==4  ShowElse=off
  Merge : Merge  Inputs=4
  Merge1 : Merge  Inputs=4
  Real Time : Subsystem
  Real Time1 : Subsystem
  T_start : Outport
  T_stop : Outport  Port=2
  wires:
  Constant/1 -> If/1
  T_min/1 -> Every Day1/1(T_min), Real Time/1(T_min), Every Day/1(T_min)
  T_max/1 -> Every Day1/2(T_max), Real Time/2(T_max), Every Day/2(T_max)
  <Temp>/1 -> Every Day/3(Te), Real Time/3(<Temp>)
  If/1 -> Every Day/Action
  If/2 -> Real Time/Action
  Merge/1 -> T_start/1
  Every Day/1(T_start) -> Merge/1
  Real Time/1(T_start) -> Merge/2
  Merge1/1 -> T_stop/1
  Real Time/2(T_stop) -> Merge1/2
  Every Day/2(T_stop) -> Merge1/1
  Real Time1/1(T_start) -> Merge/3
  Real Time1/2(T_stop) -> Merge1/3
  If/3 -> Real Time1/Action
  Every Day1/1(T_start) -> Merge/4
  Every Day1/2(T_stop) -> Merge1/4
  If/4 -> Every Day1/Action

== system D24P414_1_model02/Indoor Climate Models and Controls/Climate Model/Climate Model/Gases Exchange/Carbon Dynamics ==
  CarbonC : Inport
  MC_cc_i : Inport  Port=2
  GasComp : Inport  Port=3
  Te : Inport  Port=4
  Ventilation Rate : Inport  Port=5
  Bus Selector1 : BusSelector  OutputSignals=C_c
  Carbon Exchange Indoor-Outdoor : Subsystem
  Constant : Constant  Value=params.V
  Constant1 : Constant  Value=params.V
  Divide : Product  Inputs=/*
  Divide1 : Product  Inputs=*/
  External CO2 Concentration : Subsystem
  Scope : Scope  NumInputPorts=3
  Scope1 : Scope
  Sum1 : Sum  Inputs=|++-
  dC_c_dt : Outport
  C_ce : Outport  Port=2
  wires:
  Constant1/1 -> Divide/1
  Constant/1 -> Divide1/2
  Te/1 -> External CO2 Concentration/1(T_e)
  Sum1/1 -> dC_c_dt/1
  Carbon Exchange Indoor-Outdoor/1(MC_i_e) -> Sum1/3, Scope/3  "MC_i_e"
  Divide1/1 -> Sum1/2, Scope/2  "MC_iny"
  Divide/1 -> Sum1/1, Scope/1  "MC_v_i"
  MC_cc_i/1 -> Divide1/1
  External CO2 Concentration/1(C_ce) -> Carbon Exchange Indoor-Outdoor/3(C_ce), C_ce/1, Scope1/1  "C_ce"
  Bus Selector1/1 -> Carbon Exchange Indoor-Outdoor/2(C_c)  "<C_c>"
  GasComp/1 -> Bus Selector1/1
  CarbonC/1 -> Divide/2
  Ventilation Rate/1 -> Carbon Exchange Indoor-Outdoor/1(R_a)

== system D24P414_1_model02/Indoor Climate Models and Controls/Climate Model/Climate Model/Gases Exchange/Compute Mid Variables ==
  Gas_Conc : Inport
  Indoor Temperature : Inport  Port=2
  C_ce : Inport  Port=3
  Bus Creator : BusCreator  Inputs=12
  Constant : Constant  Value=params.int_air_speed
  Demux : Demux  Outputs=2
  Subsystem : Subsystem
  Gas : Outport
  wires:
  C_ce/1 -> Bus Creator/12  "C_ce"
  Subsystem/8(xH_sat) -> Bus Creator/11  "Xh_sat"
  Subsystem/7(p_a) -> Bus Creator/10  "p_a"
  Subsystem/5(C_w_sat_T_f) -> Bus Creator/8  "C_w_sat_T_f"
  Subsystem/4(C_w_sat_T_c) -> Bus Creator/7  "C_w_sat_T_c"
  Subsystem/6(xH) -> Bus Creator/9  "Xh"
  Demux/1 -> Bus Creator/2  "C_w"
  Constant/1 -> Bus Creator/1  "air_speed"
  Indoor Temperature/1 -> Subsystem/2(IndoorTemp)
  Demux/2 -> Bus Creator/3  "C_c"
  Subsystem/3(HRInt) -> Bus Creator/6  "HRInt"
  Subsystem/2(C_c_ppm) -> Bus Creator/5  "C_c_ppm"
  Subsystem/1(rho_i) -> Bus Creator/4  "rho_i"
  Bus Creator/1 -> Gas/1  "Gas"
  Gas_Conc/1 -> Subsystem/1(Gas_Conc), Demux/1

== system D24P414_1_model02/Indoor Climate Models and Controls/Climate Model/Climate Model/Gases Exchange/Water Dynamics ==
  GasComp : Inport
  Latent Heat : Inport  Port=2
  Condensation : Inport  Port=3
  He : Inport  Port=4
  Te : Inport  Port=5
  Ventilation Rate : Inport  Port=6
  Bus Selector : BusSelector  OutputSignals=QT,Qfog
  Bus Selector1 : BusSelector  OutputSignals=C_w
  Bus Selector2 : BusSelector  OutputSignals=QP_i_c,QP_i_f
  Minus : Sum  Inputs=+-
  Product : Product
  Subsystem : Subsystem
  Vapor Mass Balance : Subsystem
  dC_w_dt : Outport
  wires:
  Vapor Mass Balance/1(dC_w_dt) -> dC_w_dt/1
  Bus Selector2/2 -> Vapor Mass Balance/5(<QP_i_f>)  "<QP_i_f>"
  Bus Selector2/1 -> Vapor Mass Balance/4(<QP_i_c>)  "<QP_i_c>"
  Product/1 -> Vapor Mass Balance/3(MW_i_e)
  Bus Selector/2 -> Vapor Mass Balance/2(<Qfog>)  "<Qfog>"
  Subsystem/1(C_w_Te) -> Minus/2
  He/1 -> Subsystem/2(<Exterior Humidity>)
  Te/1 -> Subsystem/1(<Temperature>)
  Minus/1 -> Product/2
  Condensation/1 -> Bus Selector2/1
  Bus Selector1/1 -> Minus/1  "<C_w>"
  GasComp/1 -> Bus Selector1/1
  Bus Selector/1 -> Vapor Mass Balance/1(<QT_v_i>)  "<QT>"
  Latent Heat/1 -> Bus Selector/1
  Ventilation Rate/1 -> Product/1

== system D24P414_1_model02/Indoor Climate Models and Controls/Climate Model/Climate Model/Indoor Temperature Model/Conduction ==
  Indoor Temperature : Inport
  Bus Creator : BusCreator  Inputs=2
  Bus Selector : BusSelector  OutputSignals=Tfloor,Tsoil
  Conduction : MATLAB Function  TreatAsAtomicUnit=on
  Constant : Constant  Value=params.A_f
  Constant1 : Constant  Value=params.lam_s
  Constant2 : Constant  Value=params.l_s
  Constant3 : Constant  Value=params.T_ss
  QD : Outport
  wires:
  Constant/1 -> Conduction/3(A_f)
  Constant1/1 -> Conduction/4(lam_s)
  Constant2/1 -> Conduction/5(l_s)
  Constant3/1 -> Conduction/6(T_ss)
  Bus Selector/1 -> Conduction/1(T_f)  "<Tfloor>"
  Bus Selector/2 -> Conduction/2(T_s1)  "<Tsoil>"
  Indoor Temperature/1 -> Bus Selector/1
  Bus Creator/1 -> QD/1
  Conduction/2(QD_s12) -> Bus Creator/2
  Conduction/1(QD_sf1) -> Bus Creator/1

== system D24P414_1_model02/Indoor Climate Models and Controls/Climate Model/Climate Model/Indoor Temperature Model/Convection ==
  In Bus Element2 : Inport  PortName=ExteriorClimate  Element=Temp
  In Bus Element4 : Inport  PortName=ExteriorClimate  Element=Temp
  In Bus Element1 : Inport  PortName=ExteriorClimate  Element=Wind
  In Bus Element3 : Inport  PortName=ExteriorClimate  Element=Wind
  Windows : Inport  Port=2
  Indoor Temperature : Inport  Port=3
  QV_i : Inport  Port=4
  In Bus Element : Inport  Port=5  PortName=Gas  Element=rho_i
  In Bus Element5 : Inport  Port=5  PortName=Gas  Element=C_w
  In Bus Element6 : Inport  Port=5  PortName=Gas  Element=C_w_sat_T_c
  In Bus Element7 : Inport  Port=5  PortName=Gas  Element=C_w_sat_T_f
  Bus Creator : BusCreator  Inputs=5
  Bus Selector1 : BusSelector  OutputSignals=Tair
  Convection : Subsystem
      settings: PortSchema="{\"entries\":[{\"content\":{\"sides\":[{\"content\":{\"connectorIds\":[\"In1\",\"In2\",\"In3\",\"In4\",\"In5\"]},\"type\":\"ConnectorPlacement.EquallySpacedRectSide\",\"uuid\":\"490685c0-4e11-426f-bb8f-3f4d655c5ac7\"},{\"content\":{\"connectorIds\":[\"Out1\",\"Out2\",\"Out3\"],\"side\":\"RIGHT\"},\"type\":\"ConnectorPlacement.EquallySpacedRectSide\",\"uuid\":\"d4812e49-5d44-4dbe-a973-0d0765960a30\"},{\"content\":{\"connectorIds\":[\"In6\",\"In7\"],\"side\":\"TOP\"},\"type\":\"ConnectorPlacement.EquallySpacedRectSide\",\"uuid\":\"13a56147-4397-4d7e-8a08-f4127ff1f422\"},{\"content\":{\"connectorIds\":[\"Out4\"],\"side\":\"BOTTOM\"},\"type\":\"ConnectorPlacement.EquallySpacedRectSide\",\"uuid\":\"3700cf61-bbb7-4a7e-bcc8-2fc27ab64caf\"}]},\"type\":\"ConnectorPlacement.EquallySpacedConnector\",\"uuid\":\"ceadb976-1cc2-4430-962a-7e8db98fda5f\"}],\"packageUris\":[\"http://schema.mathworks.com/mf0/Connector/R2020b\"],\"version\":\"1.0\"}"
  Subsystem : Subsystem
      settings: PortSchema="{\"entries\":[{\"content\":{\"sides\":[{\"content\":{\"connectorIds\":[\"In1\",\"In2\",\"In3\",\"In4\"]},\"type\":\"ConnectorPlacement.EquallySpacedRectSide\",\"uuid\":\"b628b76c-815c-4d2d-bf8b-9241abf78a18\"},{\"content\":{\"connectorIds\":[\"Out1\",\"Out2\"],\"side\":\"RIGHT\"},\"type\":\"ConnectorPlacement.EquallySpacedRectSide\",\"uuid\":\"d01161a9-1f84-445a-b084-f8cb6d6fe506\"},{\"content\":{\"connectorIds\":[],\"side\":\"TOP\"},\"type\":\"ConnectorPlacement.EquallySpacedRectSide\",\"uuid\":\"e7ae8035-b56b-4ea0-80c9-470a91dd5096\"},{\"content\":{\"connectorIds\":[\"In5\"],\"side\":\"BOTTOM\"},\"type\":\"ConnectorPlacement.EquallySpacedRectSide\",\"uuid\":\"28955d4e-ecf1-4383-b712-07fa8a44f693\"}]},\"type\":\"ConnectorPlacement.EquallySpacedConnector\",\"uuid\":\"e2661f4d-c009-47a9-b3ca-7a17d9ffa541\"}],\"packageUris\":[\"http://schema.mathworks.com/mf0/Connector/R2020b\"],\"version\":\"1.0\"}"
  QV : Outport  PortDimensions=5
  QP : Outport  Port=2
  R_a : Outport  Port=3
  wires:
  In Bus Element7/1 -> Convection/3(Cw_Tf)
  In Bus Element6/1 -> Convection/2(Cw_Tc)
  Bus Creator/1 -> QV/1
  Subsystem/2(QV_i_e) -> Bus Creator/1  "QV_i_e"
  Convection/1(QV_c_e) -> Bus Creator/2
  Convection/2(QV_i_c) -> Bus Creator/3
  Convection/3(QV_i_f) -> Bus Creator/4
  QV_i/1 -> Bus Creator/5  "QV_i"
  Subsystem/1(R_a) -> R_a/1
  Windows/1 -> Subsystem/4(Windows)
  Bus Selector1/1 -> Subsystem/3(<Tair>)  "<Tair>"
  In Bus Element3/1 -> Subsystem/2(wind_speed)
  In Bus Element2/1 -> Subsystem/1(T_e)
  In Bus Element/1 -> Convection/6(rho_i), Subsystem/5(rho_i)
  In Bus Element5/1 -> Convection/7(C_w)
  In Bus Element4/1 -> Convection/4(T_e)
  In Bus Element1/1 -> Convection/5(wind_speed)
  Convection/4(QP) -> QP/1
  Indoor Temperature/1 -> Convection/1(IndoorTemp), Bus Selector1/1
